simulink model "old_diff_flatness_l_nl_online"  (R2023b)
settings: Solver=FixedStepAuto  StartTime=0.0  StopTime=15  RelTol=1e-3
model workspace (MAT data in the model file):
  kp = Simulink.Parameter
  kp.DataType = 'auto'
  kp.Complexity = 'real'
  kp.Dimensions = [0 0]
undefined symbols (not defined in the file or in its folder): obstacle_x, obstacle_y, overtake_data, overtake_time
libraries: dspsigops x7, robotmobilelib x5
settings Model: Creator=RichiRettore  LastModifiedBy=RichiRettore

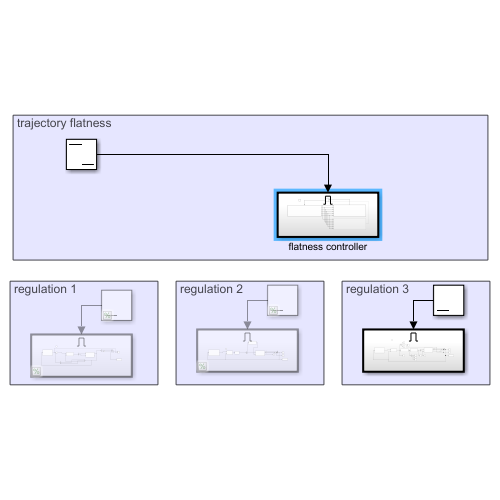
[thumbnail: Simulink's stored preview of the top-level diagram]
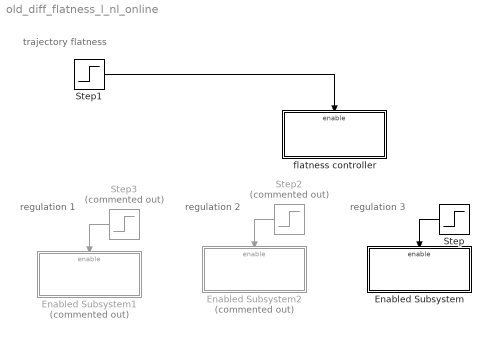
== system old_diff_flatness_l_nl_online ==
  note: regulation 3
  note: regulation 2
  note: regulation 1
  note: trajectory flatness
  Enabled Subsystem : Subsystem  TreatAsAtomicUnit=on
  Enabled Subsystem1 : Subsystem  Commented=on  TreatAsAtomicUnit=on
  Enabled Subsystem2 : Subsystem  Commented=on  TreatAsAtomicUnit=on
  Step : Step  Time=10  SampleTime=0
  Step1 : Step  Time=10  Before=1  After=0  SampleTime=0
  Step2 : Step  Commented=on  Time=10  SampleTime=0
  Step3 : Step  Commented=on  Time=10  SampleTime=0
  flatness controller : Subsystem  TreatAsAtomicUnit=on
  wires:
  Step1/1 -> flatness controller/Enable
  Step/1 -> Enabled Subsystem/Enable
  Step2/1 -> Enabled Subsystem2/Enable
  Step3/1 -> Enabled Subsystem1/Enable

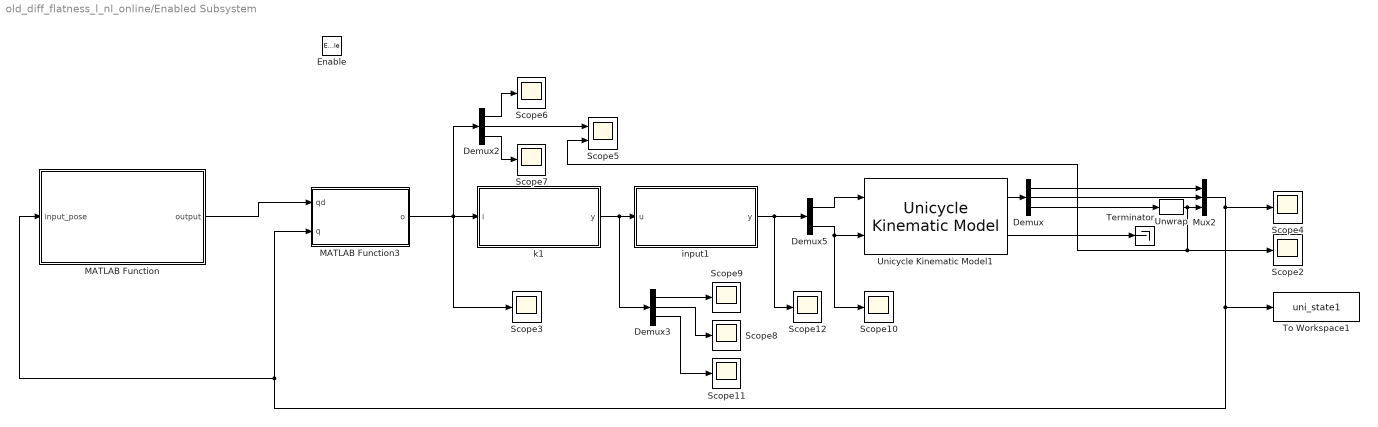
== system old_diff_flatness_l_nl_online/Enabled Subsystem ==
  Enable : EnablePort
  Demux : Demux  Outputs=3
  Demux2 : Demux  Outputs=3
  Demux3 : Demux  Outputs=3
  Demux5 : Demux  Outputs=2
  MATLAB Function : MATLAB Function  TreatAsAtomicUnit=on
  MATLAB Function3 : MATLAB Function  TreatAsAtomicUnit=on
  Mux2 : Mux  Inputs=3
  Scope{2..4,6..12} (10 alike) : Scope
  Scope5 : Scope  NumInputPorts=2
  Terminator : Terminator
  To Workspace1 : ToWorkspace  VariableName=uni_state1  SaveFormat=Structure With Time  SampleTime=0.004
  Unicycle Kinematic Model1 : robotmobilelib/Unicycle Kinematic Model  VehicleInputs=Vehicle Speed & Heading Angular Velocity  WheelRadius=2  WheelSpeedRange=[-Inf Inf]  InitialState=[125;60;0]  SimulateUsing=Interpreted execution
  Unwrap : dspsigops/Unwrap  tol=pi  InputProcessing=Columns as channels (frame based)  running=off
  input1 : MATLAB Function  TreatAsAtomicUnit=on
  k1 : MATLAB Function  TreatAsAtomicUnit=on
  wires:
  Mux2/1 -> To Workspace1/1, MATLAB Function/1(input_pose), MATLAB Function3/2(q), Scope4/1
  MATLAB Function3/1(o) -> Demux2/1, Scope3/1, k1/1(i)
  Demux2/3 -> Scope7/1
  Demux/1 -> Mux2/1
  Demux3/3 -> Scope11/1
  Demux/3 -> Unwrap/1
  Demux5/2 -> Scope10/1, Unicycle Kinematic Model1/2
  Unicycle Kinematic Model1/1 -> Demux/1
  Demux2/1 -> Scope6/1
  Demux3/2 -> Scope8/1
  Unicycle Kinematic Model1/2 -> Terminator/1
  input1/1(y) -> Scope12/1, Demux5/1
  MATLAB Function/1(output) -> MATLAB Function3/1(qd)
  Demux3/1 -> Scope9/1
  Demux/2 -> Mux2/2
  Demux2/2 -> Scope5/1
  k1/1(y) -> Demux3/1, input1/1(u)
  Unwrap/1 -> Scope2/1, Scope5/2, Mux2/3
  Demux5/1 -> Unicycle Kinematic Model1/1

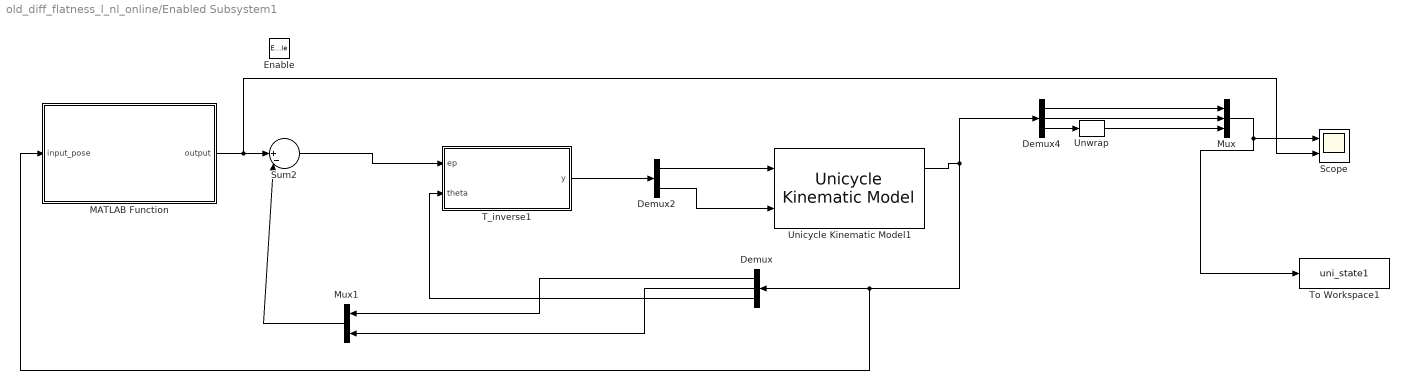
== system old_diff_flatness_l_nl_online/Enabled Subsystem1 ==
  Enable : EnablePort
  Demux : Demux  Outputs=3
  Demux2 : Demux  Outputs=2
  Demux4 : Demux  Outputs=3
  MATLAB Function : MATLAB Function  TreatAsAtomicUnit=on
  Mux : Mux  Inputs=3
  Mux1 : Mux  Inputs=2
  Scope : Scope  NumInputPorts=2
  Sum2 : Sum  Inputs=||+-|
  T_inverse1 : MATLAB Function  TreatAsAtomicUnit=on
  To Workspace1 : ToWorkspace  VariableName=uni_state1  SaveFormat=Structure With Time  SampleTime=0.001
  Unicycle Kinematic Model1 : robotmobilelib/Unicycle Kinematic Model  VehicleInputs=Vehicle Speed & Heading Angular Velocity  WheelRadius=0.1  WheelSpeedRange=[-Inf Inf]  InitialState=[125;60;0]  SimulateUsing=Interpreted execution
  Unwrap : dspsigops/Unwrap  tol=pi  InputProcessing=Columns as channels (frame based)  running=off
  wires:
  T_inverse1/1(y) -> Demux2/1
  Mux/1 -> To Workspace1/1, Scope/1
  Demux4/3 -> Unwrap/1
  Demux/1 -> Mux1/1
  Demux4/1 -> Mux/1
  Demux/3 -> T_inverse1/2(theta)
  MATLAB Function/1(output) -> Scope/2, Sum2/1
  Demux/2 -> Mux1/2
  Mux1/1 -> Sum2/2
  Demux2/2 -> Unicycle Kinematic Model1/2
  Demux2/1 -> Unicycle Kinematic Model1/1
  Unicycle Kinematic Model1/1 -> Demux4/1, MATLAB Function/1(input_pose), Demux/1
  Unwrap/1 -> Mux/3
  Sum2/1 -> T_inverse1/1(ep)
  Demux4/2 -> Mux/2

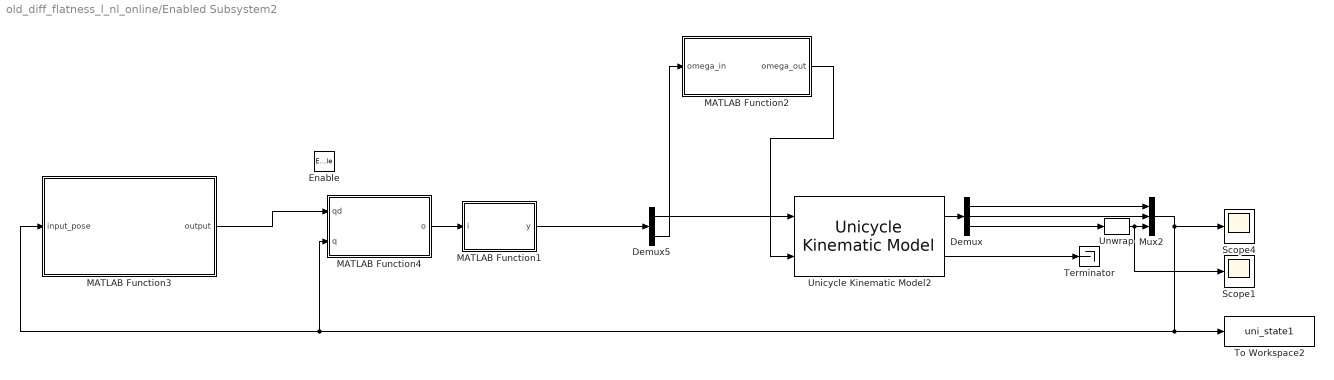
== system old_diff_flatness_l_nl_online/Enabled Subsystem2 ==
  Enable : EnablePort
  Demux : Demux  Outputs=3
  Demux5 : Demux  Outputs=2
  MATLAB Function1 : MATLAB Function  TreatAsAtomicUnit=on
  MATLAB Function2 : MATLAB Function  TreatAsAtomicUnit=on
  MATLAB Function3 : MATLAB Function  TreatAsAtomicUnit=on
  MATLAB Function4 : MATLAB Function  TreatAsAtomicUnit=on
  Mux2 : Mux  Inputs=3
  Scope1 : Scope
  Scope4 : Scope
  Terminator : Terminator
  To Workspace2 : ToWorkspace  VariableName=uni_state1  SaveFormat=Structure With Time  SampleTime=0.004
  Unicycle Kinematic Model2 : robotmobilelib/Unicycle Kinematic Model  VehicleInputs=Vehicle Speed & Heading Angular Velocity  WheelRadius=2  WheelSpeedRange=[-Inf Inf]  InitialState=[125;60;0]  SimulateUsing=Interpreted execution
  Unwrap : dspsigops/Unwrap  tol=pi  InputProcessing=Columns as channels (frame based)  running=off
  wires:
  MATLAB Function4/1(o) -> MATLAB Function1/1(i)
  Demux5/1 -> Unicycle Kinematic Model2/1
  MATLAB Function2/1(omega_out) -> Unicycle Kinematic Model2/2
  Unwrap/1 -> Scope1/1, Mux2/3
  Demux/2 -> Mux2/2
  MATLAB Function3/1(output) -> MATLAB Function4/1(qd)
  Demux/3 -> Unwrap/1
  Demux/1 -> Mux2/1
  Mux2/1 -> MATLAB Function4/2(q), MATLAB Function3/1(input_pose), To Workspace2/1, Scope4/1
  Unicycle Kinematic Model2/1 -> Demux/1
  Demux5/2 -> MATLAB Function2/1(omega_in)
  MATLAB Function1/1(y) -> Demux5/1
  Unicycle Kinematic Model2/2 -> Terminator/1

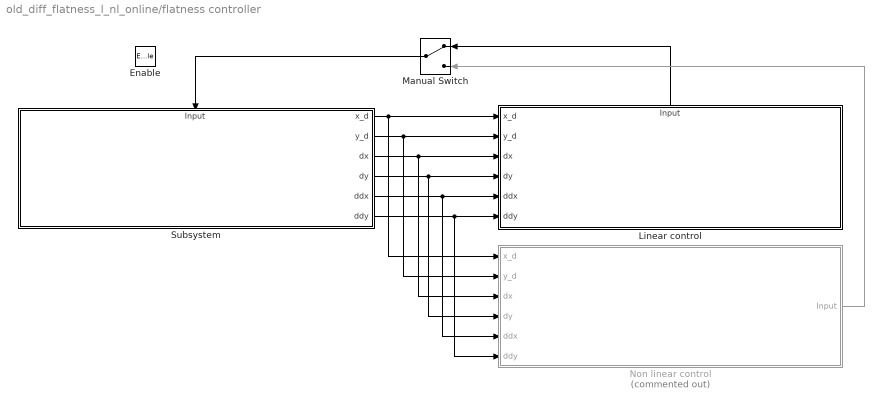
== system old_diff_flatness_l_nl_online/flatness controller ==
  Enable : EnablePort
  Linear control : Subsystem
      settings: PortSchema="{\"entries\":[{\"content\":{\"sides\":[{\"content\":{\"connectorIds\":[\"In1\",\"In2\",\"In3\",\"In4\",\"In5\",\"In6\"]},\"type\":\"ConnectorPlacement.EquallySpacedRectSide\",\"uuid\":\"9439d29c-34b2-4c3b-89f6-95a613f6df6b\"},{\"content\":{\"connectorIds\":[],\"side\":\"RIGHT\"},\"type\":\"ConnectorPlacement.EquallySpacedRectSide\",\"uuid\":\"e3292a0e-d5d9-4e7c-90ea-e2dda34ca713\"},{\"content\":{\"connectorIds\":[\"Out1\"],\"side\":\"TOP\"},\"type\":\"ConnectorPlacement.EquallySpacedRectSide\",\"uuid\":\"bc029d72-c254-41c5-9692-653abe4146db\"}]},\"type\":\"ConnectorPlacement.EquallySpacedConnector\",\"uuid\":\"066f3a1e-0ad0-413d-81a2-ec5a53f33651\"}],\"packageUris\":[\"http://schema.mathworks.com/mf0/Connector/R2020b\"],\"version\":\"1.0\"}"
  Manual Switch : ManualSwitch
  Non linear control : Subsystem  Commented=on
  Subsystem : Subsystem
      settings: PortSchema="{\"entries\":[{\"content\":{\"sides\":[{\"content\":{\"connectorIds\":[]},\"type\":\"ConnectorPlacement.EquallySpacedRectSide\",\"uuid\":\"bab0430f-2040-4f48-ad8d-487ab7428587\"},{\"content\":{\"connectorIds\":[\"Out1\",\"Out2\",\"Out3\",\"Out4\",\"Out5\",\"Out6\"],\"side\":\"RIGHT\"},\"type\":\"ConnectorPlacement.EquallySpacedRectSide\",\"uuid\":\"fe81b18b-57b7-4f8a-a498-2bb577fc7a66\"},{\"content\":{\"connectorIds\":[\"In1\"],\"side\":\"TOP\"},\"type\":\"ConnectorPlacement.EquallySpacedRectSide\",\"uuid\":\"5696e2ec-37da-4508-aed8-308f798d2cbf\"}]},\"type\":\"ConnectorPlacement.EquallySpacedConnector\",\"uuid\":\"7a90f98b-b312-4b58-9f24-f8994a9864dd\"}],\"packageUris\":[\"http://schema.mathworks.com/mf0/Connector/R2020b\"],\"version\":\"1.0\"}"
  wires:
  Linear control/1(Input) -> Manual Switch/1
  Non linear control/1(Input) -> Manual Switch/2
  Manual Switch/1 -> Subsystem/1(Input)
  Subsystem/1(x_d) -> Non linear control/1(x_d), Linear control/1(x_d)
  Subsystem/2(y_d) -> Non linear control/2(y_d), Linear control/2(y_d)
  Subsystem/3(dx) -> Non linear control/3(dx), Linear control/3(dx)
  Subsystem/4(dy) -> Non linear control/4(dy), Linear control/4(dy)
  Subsystem/5(ddx) -> Non linear control/5(ddx), Linear control/5(ddx)
  Subsystem/6(ddy) -> Non linear control/6(ddy), Linear control/6(ddy)

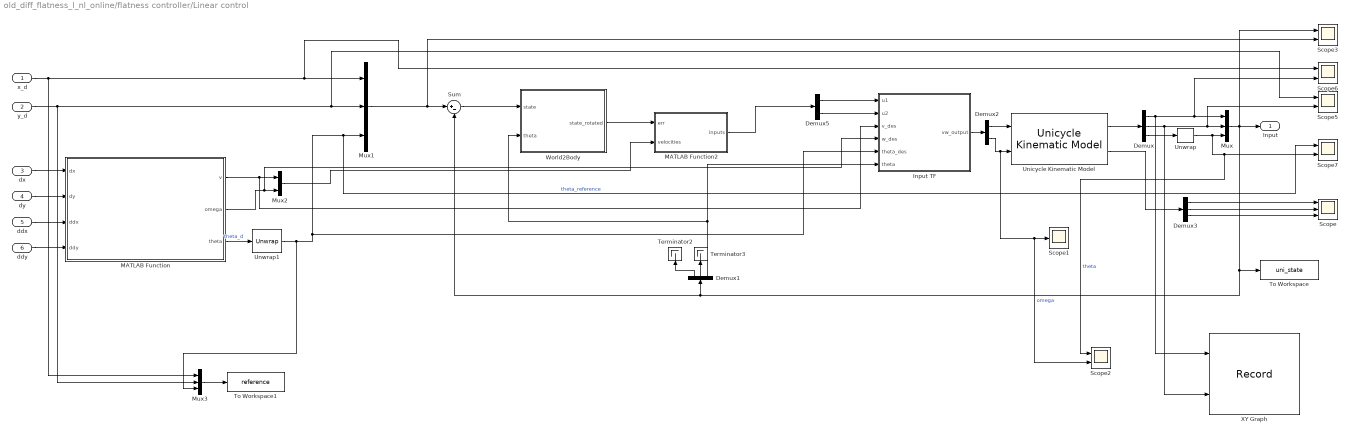
== system old_diff_flatness_l_nl_online/flatness controller/Linear control ==
  x_d : Inport
  y_d : Inport  Port=2
  dx : Inport  Port=3
  dy : Inport  Port=4
  ddx : Inport  Port=5
  ddy : Inport  Port=6
  Demux : Demux  Outputs=3
  Demux1 : Demux  Outputs=3
  Demux2 : Demux  Outputs=2
  Demux3 : Demux  Outputs=3
  Demux5 : Demux  Outputs=2
  Input TF : MATLAB Function  TreatAsAtomicUnit=on
  MATLAB Function : MATLAB Function  TreatAsAtomicUnit=on
  MATLAB Function2 : MATLAB Function  TreatAsAtomicUnit=on
  Mux : Mux  Inputs=3
  Mux1 : Mux  Inputs=3
  Mux2 : Mux  Inputs=2
  Mux3 : Mux  Inputs=3
  Scope : Scope  NumInputPorts=3
  Scope1 : Scope
  Scope{2..3,5..7} (5 alike) : Scope  NumInputPorts=2
  Sum : Sum  Inputs=|+-
  Terminator2 : Terminator
  Terminator3 : Terminator
  To Workspace : ToWorkspace  VariableName=uni_state  SaveFormat=Structure With Time  SampleTime=0.01
  To Workspace1 : ToWorkspace  VariableName=reference  SaveFormat=Structure With Time  SampleTime=0.01
  Unicycle Kinematic Model : robotmobilelib/Unicycle Kinematic Model  VehicleInputs=Vehicle Speed & Heading Angular Velocity  WheelRadius=0.1  WheelSpeedRange=[-Inf Inf]  InitialState=[125; 60; 0]  SimulateUsing=Interpreted execution
  Unwrap : dspsigops/Unwrap  tol=pi  InputProcessing=Columns as channels (frame based)  running=off
  Unwrap1 : dspsigops/Unwrap  tol=pi  InputProcessing=Columns as channels (frame based)  running=off
  World2Body : MATLAB Function  TreatAsAtomicUnit=on
  XY Graph : Record  FileSettingsInternal="{\"entries\":[{\"content\":{\"excelSettings\":{\"content\":{},\"type\":\"Streamout.ExcelSettings\"}},\"type\":\"Streamout.FileSettingStorage\",\"uuid\":\"\"}],\"packageUris\":[\"http:\\/\\/schema.mathworks.com\\/mf0\\/streamout_blocks\\/R2020a\"],\"version\":\"1.0\"}"  Layout=[1 1]  SignalsInternal="{\"entries\":[{\"content\":{\"signals\":[{\"content\":{\"blockPath\":[],\"dimensions\":[1],\"domain\":\"\",\"lineColor\":\"#a2142f\",\"port\":1,\"sid\":[\"\"],\"signalID\":516,\"signalName\":\"Demux:1\"},\"type\":\"RecordBlkView.Signal\",\"uuid\":\"\"},{\"content\":{\"blockPath\":[],\"dimensions\":[1],\"domain\":\"\",\"lineColor\":\"#139fff\",\"port\":2,\"sid\":[\"\"],\"signalID\":520,\"signalName\":\"Demux:2\"},\"type\":\"RecordBlkView.Signal\",\"uuid\":\"\"}]},\"type\":\"RecordBlkView.InputSignals\",\"uuid\":\"\"}],\"packageUris\":[\"http:\\/\\/schema.mathworks.com\\/mf0\\/streamout_blocks\\/R2020a\"],\"version\":\"1.0\"}"  VisualizationBindings="{\"xyplotplugin\":{\"info\":[{\"series\":[],\"subplotID\":1}]}}"  CompatibilityTag=XY
  Input : Outport
  wires:
  dx/1 -> MATLAB Function/1(dx)
  Demux1/3 -> Input TF/6(theta), World2Body/2(theta)
  ddx/1 -> MATLAB Function/3(ddx)
  Sum/1 -> World2Body/1(state)
  World2Body/1(state_rotated) -> MATLAB Function2/1(err)
  Demux2/1 -> Unicycle Kinematic Model/1
  Demux2/2 -> Scope2/2, Scope1/1, Unicycle Kinematic Model/2  "omega"
  Input TF/1(vw_output) -> Demux2/1
  Mux1/1 -> Scope3/2, Sum/1
  Demux/1 -> Scope6/2, Mux/1, XY Graph/1
  Mux2/1 -> MATLAB Function2/2(velocities)
  Demux/2 -> XY Graph/2, Mux/2, Scope5/2
  ddy/1 -> MATLAB Function/4(ddy)
  dy/1 -> MATLAB Function/2(dy)
  Demux1/1 -> Terminator2/1
  Demux1/2 -> Terminator3/1
  Unwrap/1 -> Scope2/1, Scope7/2, Mux/3  "theta"
  MATLAB Function/1(v) -> Input TF/3(v_des), Mux2/1
  MATLAB Function/2(omega) -> Input TF/4(w_des), Mux2/2
  MATLAB Function2/1(inputs) -> Demux5/1
  Demux5/1 -> Input TF/1(u1)
  Demux5/2 -> Input TF/2(u2)
  Mux/1 -> Scope3/1, Sum/2, Demux1/1, To Workspace/1, Input/1
  Unicycle Kinematic Model/1 -> Demux/1
  Demux/3 -> Unwrap/1
  MATLAB Function/3(theta) -> Unwrap1/1  "theta_d"
  Unicycle Kinematic Model/2 -> Demux3/1
  Demux3/1 -> Scope/1
  Demux3/2 -> Scope/2
  Demux3/3 -> Scope/3
  Mux3/1 -> To Workspace1/1
  y_d/1 -> Mux3/2, Mux1/2, Scope5/1
  Unwrap1/1 -> Mux3/3, Scope7/1, Mux1/3, Input TF/5(theta_des)  "theta_reference"
  x_d/1 -> Mux3/1, Scope6/1, Mux1/1

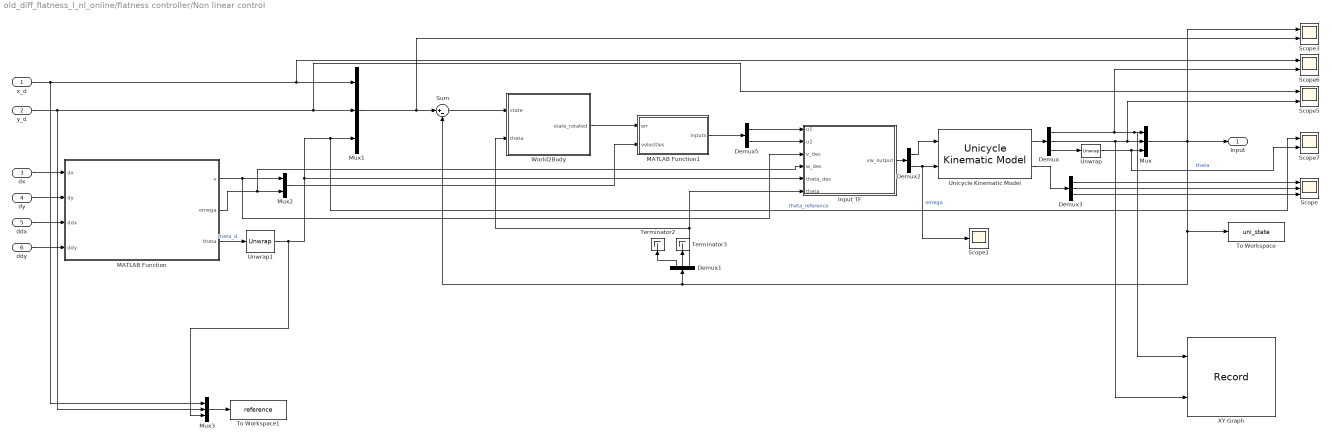
== system old_diff_flatness_l_nl_online/flatness controller/Non linear control ==
  x_d : Inport
  y_d : Inport  Port=2
  dx : Inport  Port=3
  dy : Inport  Port=4
  ddx : Inport  Port=5
  ddy : Inport  Port=6
  Demux : Demux  Outputs=3
  Demux1 : Demux  Outputs=3
  Demux2 : Demux  Outputs=2
  Demux3 : Demux  Outputs=3
  Demux5 : Demux  Outputs=2
  Input TF : MATLAB Function  TreatAsAtomicUnit=on
  MATLAB Function : MATLAB Function  TreatAsAtomicUnit=on
  MATLAB Function1 : MATLAB Function  TreatAsAtomicUnit=on
  Mux : Mux  Inputs=3
  Mux1 : Mux  Inputs=3
  Mux2 : Mux  Inputs=2
  Mux3 : Mux  Inputs=3
  Scope : Scope  NumInputPorts=3
  Scope1 : Scope
  Scope{3,5..7} (4 alike) : Scope  NumInputPorts=2
  Sum : Sum  Inputs=|+-
  Terminator2 : Terminator
  Terminator3 : Terminator
  To Workspace : ToWorkspace  VariableName=uni_state  SaveFormat=Structure With Time  SampleTime=0.01
  To Workspace1 : ToWorkspace  VariableName=reference  SaveFormat=Structure With Time  SampleTime=0.01
  Unicycle Kinematic Model : robotmobilelib/Unicycle Kinematic Model  VehicleInputs=Vehicle Speed & Heading Angular Velocity  WheelRadius=0.1  WheelSpeedRange=[-Inf Inf]  InitialState=[125; 60; 0]  SimulateUsing=Interpreted execution
  Unwrap : dspsigops/Unwrap  tol=pi  InputProcessing=Columns as channels (frame based)  running=off
  Unwrap1 : dspsigops/Unwrap  tol=pi  InputProcessing=Columns as channels (frame based)  running=off
  World2Body : MATLAB Function  TreatAsAtomicUnit=on
  XY Graph : Record  FileSettingsInternal="{\"entries\":[{\"content\":{\"excelSettings\":{\"content\":{},\"type\":\"Streamout.ExcelSettings\"}},\"type\":\"Streamout.FileSettingStorage\",\"uuid\":\"\"}],\"packageUris\":[\"http:\\/\\/schema.mathworks.com\\/mf0\\/streamout_blocks\\/R2020a\"],\"version\":\"1.0\"}"  Layout=[1 1]  SignalsInternal="{\"entries\":[{\"content\":{},\"type\":\"RecordBlkView.InputSignals\",\"uuid\":\"\"}],\"packageUris\":[\"http:\\/\\/schema.mathworks.com\\/mf0\\/streamout_blocks\\/R2020a\"],\"version\":\"1.0\"}"  VisualizationBindings="{\"xyplotplugin\":{\"info\":[{\"series\":[],\"subplotID\":1}]}}"  CompatibilityTag=XY
  Input : Outport
  wires:
  Demux5/1 -> Input TF/1(u1)
  MATLAB Function/3(theta) -> Unwrap1/1  "theta_d"
  Demux/3 -> Unwrap/1
  ddx/1 -> MATLAB Function/3(ddx)
  Demux1/2 -> Terminator3/1
  Demux/1 -> XY Graph/1, Mux/1, Scope6/2
  Mux/1 -> Sum/2, Demux1/1, To Workspace/1, Input/1, Scope3/1
  MATLAB Function/2(omega) -> Input TF/4(w_des), Mux2/2
  Demux2/2 -> Scope1/1, Unicycle Kinematic Model/2  "omega"
  y_d/1 -> Mux1/2, Scope5/1, Mux3/2
  Demux5/2 -> Input TF/2(u2)
  Demux/2 -> XY Graph/2, Scope5/2, Mux/2
  MATLAB Function/1(v) -> Mux2/1, Input TF/3(v_des)
  dx/1 -> MATLAB Function/1(dx)
  ddy/1 -> MATLAB Function/4(ddy)
  Unicycle Kinematic Model/1 -> Demux/1
  Unwrap1/1 -> Mux3/3, Scope7/1, Mux1/3, Input TF/5(theta_des)  "theta_reference"
  Mux1/1 -> Scope3/2, Sum/1
  Mux2/1 -> MATLAB Function1/2(velocities)
  dy/1 -> MATLAB Function/2(dy)
  Unwrap/1 -> Scope7/2, Mux/3  "theta"
  Input TF/1(vw_output) -> Demux2/1
  Sum/1 -> World2Body/1(state)
  Demux1/3 -> Input TF/6(theta), World2Body/2(theta)
  x_d/1 -> Mux3/1, Scope6/1, Mux1/1
  MATLAB Function1/1(inputs) -> Demux5/1
  Demux2/1 -> Unicycle Kinematic Model/1
  World2Body/1(state_rotated) -> MATLAB Function1/1(err)
  Demux1/1 -> Terminator2/1
  Unicycle Kinematic Model/2 -> Demux3/1
  Demux3/1 -> Scope/1
  Demux3/2 -> Scope/2
  Demux3/3 -> Scope/3
  Mux3/1 -> To Workspace1/1

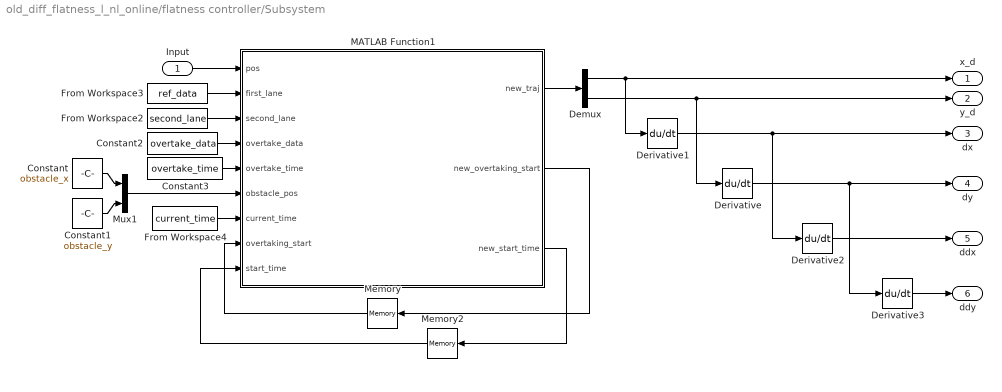
== system old_diff_flatness_l_nl_online/flatness controller/Subsystem ==
  Input : Inport
  Constant : Constant  Value=obstacle_x
  Constant1 : Constant  Value=obstacle_y
  Constant2 : Constant  Value=overtake_data
  Constant3 : Constant  Value=overtake_time
  Demux : Demux  Outputs=2
  Derivative{,1..3} (4 alike) : Derivative
  From Workspace2 : FromWorkspace  VariableName=second_lane
  From Workspace3 : FromWorkspace  VariableName=ref_data
  From Workspace4 : FromWorkspace  VariableName=current_time
  MATLAB Function1 : MATLAB Function  TreatAsAtomicUnit=on
  Memory : Memory
  Memory2 : Memory
  Mux1 : Mux  Inputs=2
  x_d : Outport
  y_d : Outport  Port=2
  dx : Outport  Port=3
  dy : Outport  Port=4
  ddx : Outport  Port=5
  ddy : Outport  Port=6
  wires:
  Derivative/1 -> dy/1, Derivative3/1
  Derivative3/1 -> ddy/1
  Derivative1/1 -> Derivative2/1, dx/1
  MATLAB Function1/1(new_traj) -> Demux/1
  Demux/1 -> x_d/1, Derivative1/1
  Demux/2 -> y_d/1, Derivative/1
  Derivative2/1 -> ddx/1
  From Workspace3/1 -> MATLAB Function1/2(first_lane)
  MATLAB Function1/3(new_start_time) -> Memory2/1
  Memory/1 -> MATLAB Function1/8(overtaking_start)
  Memory2/1 -> MATLAB Function1/9(start_time)
  MATLAB Function1/2(new_overtaking_start) -> Memory/1
  From Workspace2/1 -> MATLAB Function1/3(second_lane)
  From Workspace4/1 -> MATLAB Function1/7(current_time)
  Mux1/1 -> MATLAB Function1/6(obstacle_pos)
  Constant/1 -> Mux1/1
  Constant3/1 -> MATLAB Function1/5(overtake_time)
  Constant1/1 -> Mux1/2
  Constant2/1 -> MATLAB Function1/4(overtake_data)
  Input/1 -> MATLAB Function1/1(pos)

== matlab function old_diff_flatness_l_nl_online/Enabled Subsystem/input1 ==
  data: u input; y output
function y = fcn(u)
    v=u(2)*u(1);
    w=u(3);

    y = [v;w];

== matlab function old_diff_flatness_l_nl_online/Enabled Subsystem/k1 ==
  data: i input; y output
function y = fcn(i)
    k1=10;
    k2=40;
    k3=8;
    
    rho=i(1);
    gamma=i(2);
    delta=i(3);

    u=k1*cos(gamma);
    
    if gamma > 0.0001
        w = k2 * gamma + k1 * sin(gamma) * cos(gamma) / gamma * (gamma + k3 * delta);
    else
        w=0;
    end

    %if abs(gamma) > 0.001
    %    w = k2 * gamma + k1 * sin(gamma) * cos(gamma) / gamma * (gamma + k3 * delta);
    %else
    %    w = k2 * gamma + k1 * sin(gamma) * cos(gamma) * (k3 * delta);
    %end

    y = [rho;u;w];

== matlab function old_diff_flatness_l_nl_online/Enabled Subsystem2/MATLAB Function1 ==
  data: i input; y output
function y = fcn(i)
k1=20;
k2=30;
k3=4;
rho=i(1);
gamma=i(2);
delta=i(3);
v=k1*rho*cos(gamma);
w=k2*gamma+(k1* ((sin(gamma)*cos(gamma))/gamma) * (gamma+k3*delta));
y = [v;w];

== matlab function old_diff_flatness_l_nl_online/Enabled Subsystem2/MATLAB Function2 ==
  data: omega_in input; omega_out output
function omega_out = check_omega(omega_in)
    % Check if omega (angular velocity) is finite
    if ~isfinite(omega_in)
        omega_out = 0;  % Set omega to a default value, e.g., 0 if it is NaN or Inf
    else
        omega_out = omega_in;  % Otherwise, pass the input value
    end
end

== matlab function old_diff_flatness_l_nl_online/Enabled Subsystem2/MATLAB Function3 ==
  settings: updateMethod=DISCRETE
  data: input_pose input; output output
function output = check_and_update(input_pose)
    % Input:
    %   input_pose - a vector [x; y; theta]
    % Output:
    %   output - a vector [x_out; y_out]

    % Define the target coordinates
   
    persistent target_y; % Define target_y as persistent so it can retain its value
    persistent has_updated; % Flag to track if the update has already occurred
    persistent target_x;
    persistent target_thet;
    % Initialize persistent variables
    if isempty(target_y)
        target_y = 60; % Initial value
        target_x=270;
        target_thet=0;
    end
    if isempty(has_updated)
        has_updated = false; % Initialize the flag
    end

    % Extract x, y from input_pose
    x = input_pose(1);
    y = input_pose(2);
    theta=input_pose(3);
    tolerance = 2;

    % Check if the pose is near the target position
    if abs(x - target_x) <= tolerance && abs(y - target_y) <= tolerance && ~has_updated  && abs(theta - target_thet) <= 0.2
        % Update y-coordinate only once
        target_y = 90;
        target_x=280;
        target_thet=pi/2;
        has_updated = true; % Set the flag to prevent future updates
    end

    % Output the updated or unchanged target coordinates
    output = [target_x; target_y;target_thet];
end

== matlab function old_diff_flatness_l_nl_online/Enabled Subsystem2/MATLAB Function4 ==
  data: qd input; o output; q input
function o = fcn(qd,q)
    xi=q(1);
    yi=q(2);
    thetai=q(3);

    R = [cos(qd(3)), sin(qd(3));
        -sin(qd(3)), cos(qd(3))];
    

    x = (xi - qd(1));
    y = (yi - qd(2));
    theta = (thetai - qd(3));

    xy_new = (R * [x; y])';
    x = xy_new(1);
    y = xy_new(2);


    theta=mod(theta+pi,2*pi)-pi;

    rho=sqrt(x^2+y^2);
    gamma=atan2(y,x)+pi-theta;
    delta=gamma+theta;

    delta=mod(delta+pi,2*pi)-pi;
    gamma=mod(gamma+pi,2*pi)-pi;

    o = [rho;gamma;delta];

== matlab function old_diff_flatness_l_nl_online/Enabled Subsystem1/MATLAB Function ==
  settings: updateMethod=DISCRETE
  data: input_pose input; output output
function output = check_and_update(input_pose)
    % Input:
    %   input_pose - a vector [x; y; theta]
    % Output:
    %   output - a vector [x_out; y_out]

    % Define the target coordinates
   
    persistent target_y; % Define target_y as persistent so it can retain its value
    persistent has_updated; % Flag to track if the update has already occurred
    persistent target_x;
    % Initialize persistent variables
    if isempty(target_y)

        target_y = 60; % Initial value
        target_x=270;
    end
    if isempty(has_updated)
        has_updated = false; % Initialize the flag
    end

    % Extract x, y from input_pose
    x = input_pose(1);
    y = input_pose(2);
    tolerance = 2;

    % Check if the pose is near the target position
    if abs(x - target_x) <= tolerance && abs(y - target_y)<= tolerance && ~has_updated
        % Update y-coordinate only once

        target_y = 90;
        target_x=280;
        has_updated = true; % Set the flag to prevent future updates
    end

    % Output the updated or unchanged target coordinates
    output = [target_x; target_y];
end

== matlab function old_diff_flatness_l_nl_online/Enabled Subsystem1/T_inverse1 ==
  data: ep input; y output; theta input
function y = fcn(ep,theta)
kv=40;
kw=50;
v=kv*(ep(1)*cos(theta)+ep(2)*sin(theta));
w=kw*(atan2(-ep(2),-ep(1))+pi-theta);
y = [v;w];

== matlab function old_diff_flatness_l_nl_online/flatness controller/Subsystem/MATLAB Function1 ==
  data: pos input; first_lane input; new_traj output; second_lane input; overtake_data input; overtake_time input; obstacle_pos input size=[2]; current_time input; overtaking_start input; new_overtaking_start output; new_start_time output; start_time input
function [new_traj, new_overtaking_start, new_start_time]  = fcn(pos,first_lane, second_lane, overtake_data, overtake_time, obstacle_pos, current_time, overtaking_start, start_time)

detection_margin_x = 85; % Detection range in x-direction
detection_margin_y = 55; % Detection range in y-direction
early_detection_distance = 60; % Distance ahead of obstacle to start overtaking

% Check if obstacle is within detection range and ahead of the obstacle   
if ~overtaking_start   
    if (abs(pos(1) - obstacle_pos(1)) < detection_margin_x && abs(pos(2) - obstacle_pos(2)) < detection_margin_y) && pos(1) < obstacle_pos(1) + early_detection_distance
        new_overtaking_start = 1;
        new_start_time = current_time;
    else
        new_overtaking_start = overtaking_start;
        new_start_time = start_time;
    end
    idx = 1;
else
    idx = find(abs(overtake_time - (current_time - start_time)) <= 1e-3, 1);
    if ~isempty(idx)
        new_overtaking_start = overtaking_start;
    else
        new_overtaking_start = 0;
        idx = 1;
    end
    new_start_time = start_time;
end

new_traj = first_lane + (second_lane-first_lane)*overtake_data(idx);

== matlab function old_diff_flatness_l_nl_online/flatness controller/Non linear control/MATLAB Function1 ==
  data: err input; velocities input; inputs output
function inputs = fcn(err , velocities)
    d = 1 / sqrt(2);
    b = 10;
    vd = velocities(1);
    wd = velocities(2);
    e3 = err(3);

    % Safeguard for small ed
    e3 = sign(e3) * max(abs(e3), 1e-4);
    
    % Gains
    k1 = 2 * d * sqrt(b*vd+wd^2);
    k2 = b;
    k3 = k1;

    % Clamp kf to avoid large values
    kf = k2*vd*(sin(e3)/e3);
    max_kf = 800;
    kf = max(min(kf, max_kf), -max_kf);

    % Gain matrix
    k = [-k1, 0, 0;
         0, -kf, -k3];
    
    % Compute inputs
    inputs = k * err;
end

== matlab function old_diff_flatness_l_nl_online/flatness controller/Linear control/World2Body ==
  data: state input; state_rotated output; theta input
function state_rotated = rotation_matrix(state, theta)
% ROTATION_MATRIX Rotates the position [x; y] by an input angle theta.
%
% Inputs:
%   state - 3x1 vector representing [x; y; theta_state]
%   theta - Rotation angle in radians (scalar)
%
% Outputs:
%   state_rotated - 3x1 vector representing the rotated state [x_rot; y_rot; theta_state]

    % Extract x, y, and theta_state from the input state
    x = state(1);
    y = state(2);
    theta_state = state(3);

    % 2D rotation matrix for the x and y components
    R = [cos(theta), sin(theta);
         -sin(theta),  cos(theta)];

    % Rotate the [x; y] part of the state
    xy_rotated = R * [x; y];

    % Combine the rotated x, y, and the original theta_state into a 3x1 vector
    state_rotated = [xy_rotated; theta_state];
end

== matlab function old_diff_flatness_l_nl_online/flatness controller/Linear control/MATLAB Function ==
  data: v output; omega output; theta output; dx input; dy input; ddx input; ddy input
function [v, omega, theta] = unicycle_flatness_num(dx, dy, ddx, ddy)
    % Compute linear velocity safely
    velocity_magnitude = sqrt(dx^2 + dy^2);
    if velocity_magnitude < 1e-4
        v = sign(velocity_magnitude)*1e-4;
    else
        v = velocity_magnitude;
    end
    % Compute heading angle
    theta = atan2(dy, dx);

    % Compute angular velocity safely
    denominator = v^2;
    if denominator < 1e-4
        omega = (dx * ddy - dy * ddx) / 1e-4;
    else
        omega = (dx * ddy - dy * ddx) / denominator;
    end
end

== matlab function old_diff_flatness_l_nl_online/flatness controller/Linear control/Input TF ==
  data: u1 input; u2 input; v_des input; w_des input; theta_des input; vw_output output; theta input
function vw_output = input_transformation(u1,u2, v_des,w_des,theta_des, theta)
% INPUT_TRANSFORMATION Computes the transformed velocities v and w.
%
% Inputs:
%   u        - 2x1 vector [u1; u2]
%   vwt_des  - 3x1 vector [v_des; w_des; theta_des]
%   theta    - Scalar rotation angle in radians
%
% Outputs:
%   vw_output - 2x1 vector [v; w] representing the transformed velocities
 
    
    % Compute the transformed velocities
    v = v_des * cos(theta_des - theta) - u1;
    w = w_des - u2;

    % Combine into a 2x1 output vector
    vw_output = [v; w];
end

== matlab function old_diff_flatness_l_nl_online/flatness controller/Linear control/MATLAB Function2 ==
  data: err input; velocities input; inputs output
function inputs = fcn(err , velocities)
    d = 1 / (sqrt(2));
    a = 200;
    vd = velocities(1);
    wd = velocities(2);
    
    % Gains
    k1 = 2 * d * a;
    k2 = (a^2 - wd^2) / vd;
    k3 = k1;
    
    % Clamp k2 to avoid large values
    max_k2 = 1000;
    k2 = min(k2, max_k2);
    
    % Gain matrix
    k = [-k1, 0, 0;
         0, -k2, -k3];
    
    % Compute inputs
    inputs = k * err;
end

== matlab function old_diff_flatness_l_nl_online/flatness controller/Non linear control/Input TF ==
  data: u1 input; u2 input; v_des input; w_des input; theta_des input; vw_output output; theta input
function vw_output = input_transformation(u1,u2, v_des,w_des,theta_des, theta)
% INPUT_TRANSFORMATION Computes the transformed velocities v and w.
%
% Inputs:
%   u        - 2x1 vector [u1; u2]
%   vwt_des  - 3x1 vector [v_des; w_des; theta_des]
%   theta    - Scalar rotation angle in radians
%
% Outputs:
%   vw_output - 2x1 vector [v; w] representing the transformed velocities
 
    
    % Compute the transformed velocities
    v = v_des * cos(theta_des - theta) - u1;
    w = w_des - u2;

    % Combine into a 2x1 output vector
    vw_output = [v; w];
end

== matlab function old_diff_flatness_l_nl_online/flatness controller/Non linear control/MATLAB Function ==
  data: v output; omega output; theta output; dx input; dy input; ddx input; ddy input
function [v, omega, theta] = unicycle_flatness_num(dx, dy, ddx, ddy)
    % Compute linear velocity safely
    velocity_magnitude = sqrt(dx^2 + dy^2);
    if velocity_magnitude < 1e-4
        v = sign(velocity_magnitude)*1e-4;
    else
        v = velocity_magnitude;
    end
    % Compute heading angle
    theta = atan2(dy, dx);

    % Compute angular velocity safely
    denominator = v^2;
    if denominator < 1e-4
        omega = (dx * ddy - dy * ddx) / 1e-4;
    else
        omega = (dx * ddy - dy * ddx) / denominator;
    end
end

== matlab function old_diff_flatness_l_nl_online/Enabled Subsystem/MATLAB Function ==
  settings: updateMethod=DISCRETE
  data: input_pose input; output output
function output = check_and_update(input_pose)
    % Input:
    %   input_pose - a vector [x; y; theta]
    % Output:
    %   output - a vector [x_out; y_out]

    % Define the target coordinates
   
    persistent target_y; % Define target_y as persistent so it can retain its value
    persistent has_updated; % Flag to track if the update has already occurred
    persistent target_x;
    persistent target_thet;
    % Initialize persistent variables
    if isempty(target_y)
        target_y = 60; % Initial value
        target_x=270;
        target_thet=0;
    end
    if isempty(has_updated)
        has_updated = false; % Initialize the flag
    end

    % Extract x, y from input_pose
    x = input_pose(1);
    y = input_pose(2);
    theta=input_pose(3);
    tolerance = 2;

    % Check if the pose is near the target position
    if abs(x - target_x) <= tolerance && abs(y - target_y) <= tolerance && ~has_updated  && abs(theta - target_thet) <= 0.2
        % Update y-coordinate only once
        target_y = 90;
        target_x=280;
        target_thet=pi/2;
        has_updated = true; % Set the flag to prevent future updates
    end

    % Output the updated or unchanged target coordinates
    output = [target_x; target_y;target_thet];
end

== matlab function old_diff_flatness_l_nl_online/flatness controller/Non linear control/World2Body ==
  data: state input; state_rotated output; theta input
function state_rotated = rotation_matrix(state, theta)
% ROTATION_MATRIX Rotates the position [x; y] by an input angle theta.
%
% Inputs:
%   state - 3x1 vector representing [x; y; theta_state]
%   theta - Rotation angle in radians (scalar)
%
% Outputs:
%   state_rotated - 3x1 vector representing the rotated state [x_rot; y_rot; theta_state]

    % Extract x, y, and theta_state from the input state
    x = state(1);
    y = state(2);
    theta_state = state(3);

    % 2D rotation matrix for the x and y components
    R = [cos(theta), sin(theta);
         -sin(theta),  cos(theta)];

    % Rotate the [x; y] part of the state
    xy_rotated = R * [x; y];

    % Combine the rotated x, y, and the original theta_state into a 3x1 vector
    state_rotated = [xy_rotated; theta_state];
end

== matlab function old_diff_flatness_l_nl_online/Enabled Subsystem/MATLAB Function3 ==
  data: qd input; o output; q input
function o = fcn(qd,q)
    xi=q(1);
    yi=q(2);
    thetai=q(3);

    R = [cos(qd(3)), sin(qd(3));
        -sin(qd(3)), cos(qd(3))];
    

    x = (xi - qd(1));
    y = (yi - qd(2));
    theta = (thetai - qd(3));

    xy_new = (R * [x; y])';
    x = xy_new(1);
    y = xy_new(2);


    theta=mod(theta+pi,2*pi)-pi;

    rho=sqrt(x^2+y^2);
    gamma=atan2(y,x)+pi-theta;
    delta=gamma+theta;

    delta=mod(delta+pi,2*pi)-pi;
    gamma=mod(gamma+pi,2*pi)-pi;

    o = [rho;gamma;delta];
